simulink model "Zad1"  (R2023a)
settings: Solver=VariableStepAuto  StartTime=0.0  StopTime=100.0  RelTol=1e-3
model workspace (MAT data in the model file):
  K = Simulink.Parameter
  K.Value = 1
  K.DataType = 'auto'
  K.Complexity = 'real'
  K.Dimensions = [1 1]
  T1 = Simulink.Parameter
  T1.Value = 9
  T1.DataType = 'auto'
  T1.Complexity = 'real'
  T1.Dimensions = [1 1]
  T2 = Simulink.Parameter
  T2.Value = 8
  T2.DataType = 'auto'
  T2.Complexity = 'real'
  T2.Dimensions = [1 1]
  a1 = Simulink.Parameter
  a1.Value = -0.8
  a1.DataType = 'auto'
  a1.Complexity = 'real'
  a1.Dimensions = [1 1]
  a2 = Simulink.Parameter
  a2.Value = -0.86
  a2.DataType = 'auto'
  a2.Complexity = 'real'
  a2.Dimensions = [1 1]
  a3 = Simulink.Parameter
  a3.Value = -0.41
  a3.DataType = 'auto'
  a3.Complexity = 'real'
  a3.Dimensions = [1 1]
  a4 = Simulink.Parameter
  a4.Value = -0.41
  a4.DataType = 'auto'
  a4.Complexity = 'real'
  a4.Dimensions = [1 1]
values from neighbouring files (symbols this model uses):
  a1 = -0.8    [zad10.m]    (also in zad2.m; zad3.m)
  a2 = -0.86    [zad10.m]    (also in zad2.m; zad3.m)
  a3 = -0.41    [zad10.m]    (also in zad2.m; zad3.m)
  a4 = -0.41    [zad10.m]    (also in zad2.m; zad3.m)
  K = 1    [zad10.m]    (also in zad2.m; zad3.m)
  T1 = 9    [zad10.m]
  T2 = 8    [zad10.m]
settings Model: Creator=pkutyl  LastModifiedBy=pkutyl

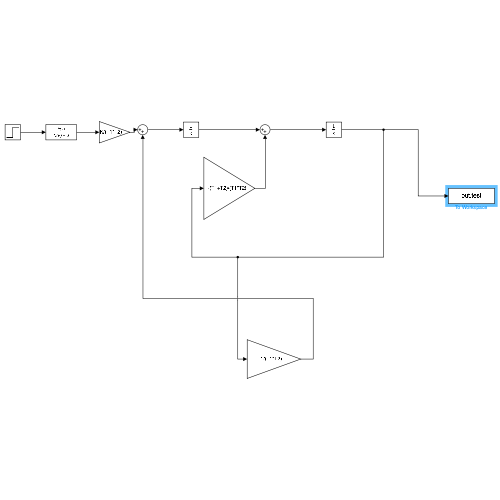
[thumbnail: Simulink's stored preview of the top-level diagram]
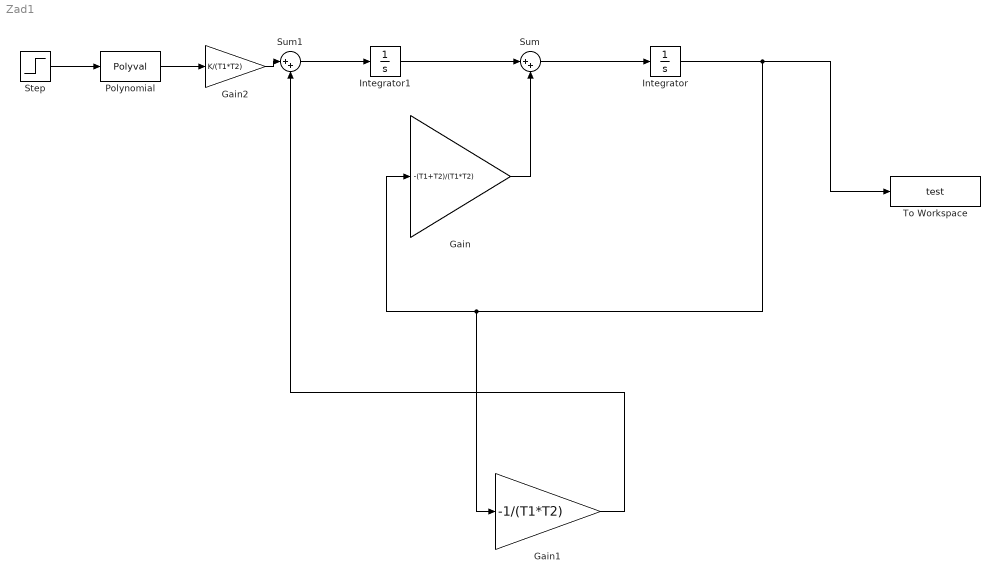
== system Zad1 ==
  Gain : Gain  Gain=-(T1+T2)/(T1*T2)
  Gain1 : Gain  Gain=-1/(T1*T2)
  Gain2 : Gain  Gain=K/(T1*T2)
  Integrator : Integrator
  Integrator1 : Integrator
  Polynomial : Polyval  Coefs=[a4,a3,a2,a1]
  Step : Step  SampleTime=0
  Sum : Sum  Inputs=|++
  Sum1 : Sum  Inputs=|++
  To Workspace : ToWorkspace  VariableName=test  SaveFormat=Structure With Time  SampleTime=-1
  wires:
  Integrator/1 -> Gain1/1, Gain/1, To Workspace/1
  Integrator1/1 -> Sum/1
  Sum/1 -> Integrator/1
  Gain/1 -> Sum/2
  Sum1/1 -> Integrator1/1
  Step/1 -> Polynomial/1
  Gain1/1 -> Sum1/2
  Polynomial/1 -> Gain2/1
  Gain2/1 -> Sum1/1
